simulink model "EVTOL_6DOF_Sim_Wrapper"  (R2025b)
settings: Solver=VariableStepAuto  StartTime=startTime  StopTime=stopTime  RelTol=1e-3
undefined symbols (not defined in the file): accel_mem_init, controller_mode, controller_sample_time, DiscIntNeverNeededParam, eul_init, gains, K_lqr_cruise, lla_init, MixMatrix, omega_init, pos_init, sat, sensor_accel_bias, sensor_accel_sigma, sensor_airdata_bias, sensor_airdata_sigma, sensor_att_bias, sensor_att_sigma, sensor_gps_posBias, sensor_gps_posSigma, sensor_gyro_bias, sensor_gyro_sigma, sensor_mag_bias, sensor_mag_sigma, sensor_magField_NED, sensor_sample_time, sensor_seed_accel, sensor_seed_airdata, sensor_seed_att, sensor_seed_gpsPos, sensor_seed_gyro, sensor_seed_mag, U_trim_lqr, useCMDs, V_mem_init, x_trim_lqr
settings Model: Creator=zbrown  LastModifiedBy=jacks

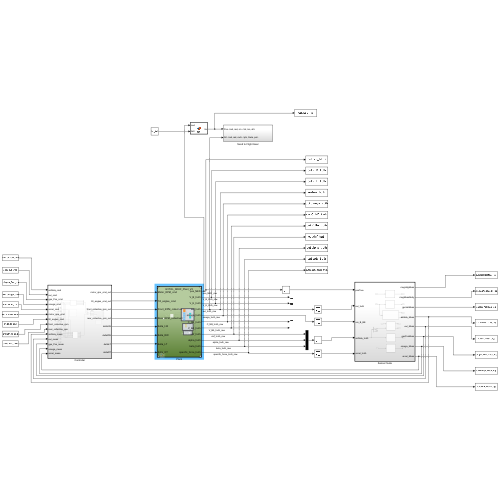
[thumbnail: Simulink's stored preview of the top-level diagram]
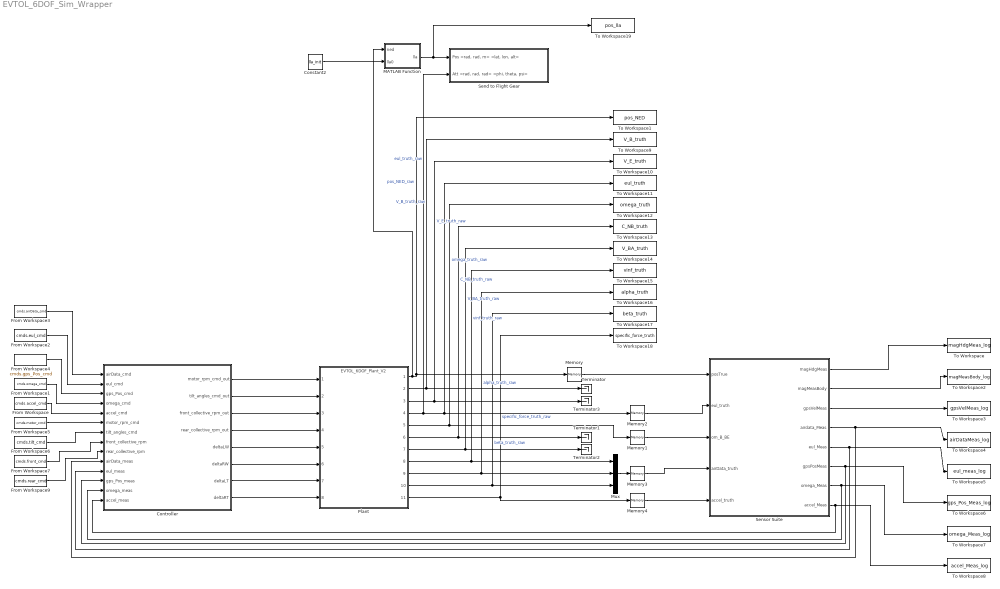
== system EVTOL_6DOF_Sim_Wrapper ==
  Constant2 : Constant  Value=lla_init
  Controller : Subsystem  TreatAsAtomicUnit=on  SystemSampleTime=controller_sample_time
  From Workspace : FromWorkspace  VariableName=cmds.accel_cmd
  From Workspace1 : FromWorkspace  VariableName=cmds.omega_cmd
  From Workspace2 : FromWorkspace  VariableName=cmds.eul_cmd
  From Workspace3 : FromWorkspace  VariableName=cmds.airData_cmd
  From Workspace4 : FromWorkspace  VariableName=cmds.gps_Pos_cmd
  From Workspace5 : FromWorkspace  VariableName=cmds.motor_cmd
  From Workspace6 : FromWorkspace  VariableName=cmds.tilt_cmd
  From Workspace7 : FromWorkspace  VariableName=cmds.front_cmd
  From Workspace9 : FromWorkspace  VariableName=cmds.rear_cmd
  MATLAB Function : MATLAB Function  TreatAsAtomicUnit=on
  Memory : Memory  InitialCondition=pos_init
  Memory1 : Memory  InitialCondition=omega_init
  Memory2 : Memory  InitialCondition=eul_init
  Memory3 : Memory  InitialCondition=V_mem_init
  Memory4 : Memory  InitialCondition=accel_mem_init
  Mux : Mux  Inputs=3
  Plant : ModelReference  ModelNameDialog=EVTOL_6DOF_Plant_V2.slx  SimulationMode=Normal  ModelReferenceVersion=1.34
  Send to Flight Gear : Subsystem
  Sensor Suite : Subsystem  TreatAsAtomicUnit=on  SystemSampleTime=sensor_sample_time
  Terminator{,1..3} (4 alike) : Terminator
  To Workspace : ToWorkspace  VariableName=magHdgMeas_log  SaveFormat=Structure With Time  SampleTime=-1
  To Workspace1 : ToWorkspace  VariableName=pos_NED  SaveFormat=Structure With Time  SampleTime=-1
  To Workspace10 : ToWorkspace  VariableName=V_E_truth  SaveFormat=Structure With Time  SampleTime=-1
  To Workspace11 : ToWorkspace  VariableName=eul_truth  SaveFormat=Structure With Time  SampleTime=-1
  To Workspace12 : ToWorkspace  VariableName=omega_truth  SaveFormat=Structure With Time  SampleTime=-1
  To Workspace13 : ToWorkspace  VariableName=C_NB_truth  SaveFormat=Structure With Time  SampleTime=-1
  To Workspace14 : ToWorkspace  VariableName=V_BA_truth  SaveFormat=Structure With Time  SampleTime=-1
  To Workspace15 : ToWorkspace  VariableName=vinf_truth  SaveFormat=Structure With Time  SampleTime=-1
  To Workspace16 : ToWorkspace  VariableName=alpha_truth  SaveFormat=Structure With Time  SampleTime=-1
  To Workspace17 : ToWorkspace  VariableName=beta_truth  SaveFormat=Structure With Time  SampleTime=-1
  To Workspace18 : ToWorkspace  VariableName=specific_force_truth  SaveFormat=Structure With Time  SampleTime=-1
  To Workspace19 : ToWorkspace  VariableName=pos_lla  SaveFormat=Structure With Time  SampleTime=-1
  To Workspace2 : ToWorkspace  VariableName=magMeasBody_log  SaveFormat=Structure With Time  SampleTime=-1
  To Workspace3 : ToWorkspace  VariableName=gpsVelMeas_log  SaveFormat=Structure With Time  SampleTime=-1
  To Workspace4 : ToWorkspace  VariableName=airDataMeas_log  SaveFormat=Structure With Time  SampleTime=-1
  To Workspace5 : ToWorkspace  VariableName=eul_meas_log  SaveFormat=Structure With Time  SampleTime=-1
  To Workspace6 : ToWorkspace  VariableName=gps_Pos_Meas_log  SaveFormat=Structure With Time  SampleTime=-1
  To Workspace7 : ToWorkspace  VariableName=omega_Meas_log  SaveFormat=Structure With Time  SampleTime=-1
  To Workspace8 : ToWorkspace  VariableName=accel_Meas_log  SaveFormat=Structure With Time  SampleTime=-1
  To Workspace9 : ToWorkspace  VariableName=V_B_truth  SaveFormat=Structure With Time  SampleTime=-1
  wires:
  Plant/1 -> MATLAB Function/1(ned), Memory/1, To Workspace1/1  "pos_NED_raw"
  Plant/2 -> Terminator/1, To Workspace9/1  "V_B_truth_raw"
  Plant/3 -> Terminator3/1, To Workspace10/1  "V_E_truth_raw"
  Plant/4 -> Send to Flight Gear/2("Att <rad, rad, rad> <phi, theta, psi>"), To Workspace11/1, Memory2/1  "eul_truth_raw"
  Plant/5 -> Memory1/1, To Workspace12/1  "omega_truth_raw"
  Plant/6 -> Terminator1/1, To Workspace13/1  "C_NB_truth_raw"
  Plant/7 -> Terminator2/1, To Workspace14/1  "V_BA_truth_raw"
  Plant/8 -> Mux/1, To Workspace15/1  "vinf_truth_raw"
  Plant/9 -> Mux/2, To Workspace16/1  "alpha_truth_raw"
  Plant/10 -> Mux/3, To Workspace17/1  "beta_truth_raw"
  Plant/11 -> Memory4/1, To Workspace18/1  "specific_force_truth_raw"
  MATLAB Function/1(lla) -> To Workspace19/1, Send to Flight Gear/1("Pos <rad, rad, m> <lat, lon, alt>")
  Constant2/1 -> MATLAB Function/2(lla0)
  Mux/1 -> Memory3/1
  Controller/5(deltaLW) -> Plant/5
  Controller/6(deltaRW) -> Plant/6
  Controller/7(deltaLT) -> Plant/7
  Controller/8(deltaRT) -> Plant/8
  Controller/4(rear_collective_rpm_out) -> Plant/4
  Controller/3(front_collective_rpm_out) -> Plant/3
  Controller/2(tilt_angles_cmd_out) -> Plant/2
  Controller/1(motor_rpm_cmd_out) -> Plant/1
  Sensor Suite/8(accel_Meas) -> Controller/14(accel_meas), To Workspace8/1
  Sensor Suite/7(omega_Meas) -> To Workspace7/1, Controller/13(omega_meas)
  Sensor Suite/6(gpsPosMeas) -> Controller/12(gps_Pos_meas), To Workspace6/1
  Sensor Suite/5(eul_Meas) -> Controller/11(eul_meas), To Workspace5/1
  Sensor Suite/4(airdata_Meas) -> Controller/10(airData_meas), To Workspace4/1
  From Workspace3/1 -> Controller/1(airData_cmd)
  From Workspace2/1 -> Controller/2(eul_cmd)
  From Workspace4/1 -> Controller/3(gps_Pos_cmd)
  From Workspace1/1 -> Controller/4(omega_cmd)
  From Workspace/1 -> Controller/5(accel_cmd)
  From Workspace5/1 -> Controller/6(motor_rpm_cmd)
  From Workspace6/1 -> Controller/7(tilt_angles_cmd)
  From Workspace7/1 -> Controller/8(front_collective_rpm)
  From Workspace9/1 -> Controller/9(rear_collective_rpm)
  Sensor Suite/1(magHdgMeas) -> To Workspace/1
  Sensor Suite/2(magMeasBody) -> To Workspace2/1
  Sensor Suite/3(gpsVelMeas) -> To Workspace3/1
  Memory/1 -> Sensor Suite/1(posTrue)
  Memory4/1 -> Sensor Suite/5(accel_truth)
  Memory3/1 -> Sensor Suite/4(airData_truth)
  Memory2/1 -> Sensor Suite/2(eul_truth)
  Memory1/1 -> Sensor Suite/3(om_B_BE)

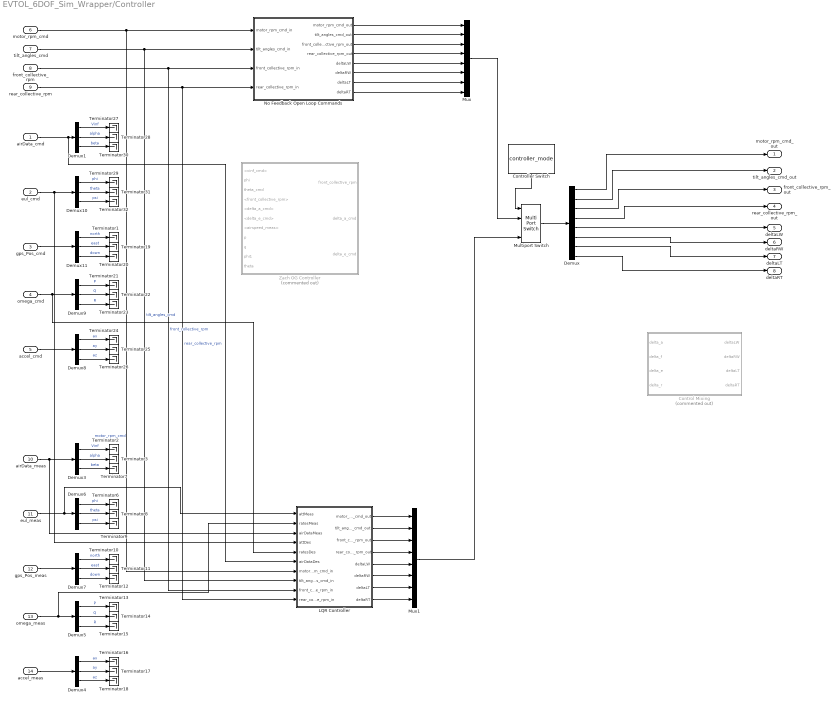
== system EVTOL_6DOF_Sim_Wrapper/Controller ==
  airData_cmd : Inport
  eul_cmd : Inport  Port=2
  gps_Pos_cmd : Inport  Port=3
  omega_cmd : Inport  Port=4
  accel_cmd : Inport  Port=5
  motor_rpm_cmd : Inport  Port=6
  tilt_angles_cmd : Inport  Port=7
  front_collective_rpm : Inport  Port=8
  rear_collective_rpm : Inport  Port=9
  airData_meas : Inport  Port=10
  eul_meas : Inport  Port=11
  gps_Pos_meas : Inport  Port=12
  omega_meas : Inport  Port=13
  accel_meas : Inport  Port=14
  Control Mixing : Subsystem  Commented=on
  Controller Switch : Constant  Value=controller_mode
  Demux : Demux  Outputs=8
  Demux{1,3..11} (10 alike) : Demux  Outputs=3
  LQR Controller : Subsystem
  Multiport Switch : MultiPortSwitch  SaturateOnIntegerOverflow=off  InputSameDT=off
  Mux : Mux  Inputs=8
  Mux1 : Mux  Inputs=8
  No Feedback Open Loop Commands : Subsystem
  Terminator{1..3,6..32} (30 alike) : Terminator
  Zach OG Controller : Subsystem  Commented=on
  motor_rpm_cmd_out : Outport
  tilt_angles_cmd_out : Outport  Port=2
  front_collective_rpm_out : Outport  Port=3
  rear_collective_rpm_out : Outport  Port=4
  deltaLW : Outport  Port=5
  deltaRW : Outport  Port=6
  deltaLT : Outport  Port=7
  deltaRT : Outport  Port=8
  wires:
  Demux11/2 -> Terminator19/1  "east"
  Demux6/3 -> Terminator9/1  "psi"
  Demux9/1 -> Terminator21/1  "P"
  motor_rpm_cmd/1 -> LQR Controller/7(motor_rpm_cmd_in), No Feedback Open Loop Commands/1(motor_rpm_cmd_in)  "motor_rpm_cmd"
  omega_cmd/1 -> LQR Controller/5(ratesDes), Demux9/1
  No Feedback Open Loop Commands/7(deltaLT) -> Mux/7
  Demux4/2 -> Terminator17/1  "ay"
  gps_Pos_cmd/1 -> Demux11/1
  Demux3/3 -> Terminator7/1  "beta"
  eul_meas/1 -> LQR Controller/1(attMeas), Demux6/1
  tilt_angles_cmd/1 -> LQR Controller/8(tilt_angles_cmd_in), No Feedback Open Loop Commands/2(tilt_angles_cmd_in)  "tilt_angles_cmd"
  Demux4/3 -> Terminator18/1  "az"
  Demux9/3 -> Terminator23/1  "R"
  airData_meas/1 -> LQR Controller/3(airDataMeas), Demux3/1
  Demux/2 -> tilt_angles_cmd_out/1
  Demux/4 -> rear_collective_rpm_out/1
  Demux8/1 -> Terminator24/1  "ax"
  Demux5/1 -> Terminator13/1  "P"
  Demux/1 -> motor_rpm_cmd_out/1
  No Feedback Open Loop Commands/6(deltaRW) -> Mux/6
  eul_cmd/1 -> LQR Controller/4(attDes), Demux10/1
  Demux3/2 -> Terminator3/1  "alpha"
  Demux9/2 -> Terminator22/1  "Q"
  Demux4/1 -> Terminator16/1  "ax"
  front_collective_rpm/1 -> LQR Controller/9(front_collective_rpm_in), No Feedback Open Loop Commands/3(front_collective_rpm_in)  "front_collective_rpm"
  Demux10/1 -> Terminator29/1  "phi"
  Demux8/3 -> Terminator26/1  "az"
  Demux7/1 -> Terminator10/1  "north"
  No Feedback Open Loop Commands/3(front_collective_rpm_out) -> Mux/3
  Demux6/1 -> Terminator6/1  "phi"
  Demux1/1 -> Terminator27/1  "Vinf"
  airData_cmd/1 -> LQR Controller/6(airDataDes), Demux1/1
  rear_collective_rpm/1 -> LQR Controller/10(rear_collective_rpm_in), No Feedback Open Loop Commands/4(rear_collective_rpm_in)  "rear_collective_rpm"
  Demux11/3 -> Terminator20/1  "down"
  Demux3/1 -> Terminator2/1  "Vinf"
  Demux6/2 -> Terminator8/1  "theta"
  Demux10/3 -> Terminator32/1  "psi"
  Demux5/3 -> Terminator15/1  "R"
  Mux/1 -> Multiport Switch/2
  No Feedback Open Loop Commands/2(tilt_angles_cmd_out) -> Mux/2
  accel_meas/1 -> Demux4/1
  No Feedback Open Loop Commands/4(rear_collective_rpm_out) -> Mux/4
  Demux5/2 -> Terminator14/1  "Q"
  Demux11/1 -> Terminator1/1  "north"
  Demux8/2 -> Terminator25/1  "ay"
  Demux1/3 -> Terminator30/1  "beta"
  gps_Pos_meas/1 -> Demux7/1
  Demux7/2 -> Terminator11/1  "east"
  Demux/3 -> front_collective_rpm_out/1
  Demux10/2 -> Terminator31/1  "theta"
  No Feedback Open Loop Commands/1(motor_rpm_cmd_out) -> Mux/1
  omega_meas/1 -> LQR Controller/2(ratesMeas), Demux5/1
  Demux7/3 -> Terminator12/1  "down"
  accel_cmd/1 -> Demux8/1
  No Feedback Open Loop Commands/8(deltaRT) -> Mux/8
  Multiport Switch/1 -> Demux/1
  No Feedback Open Loop Commands/5(deltaLW) -> Mux/5
  Demux1/2 -> Terminator28/1  "alpha"
  Controller Switch/1 -> Multiport Switch/1
  Demux/5 -> deltaLW/1
  Demux/6 -> deltaRW/1
  Demux/7 -> deltaLT/1
  Demux/8 -> deltaRT/1
  LQR Controller/7(deltaLT) -> Mux1/7
  LQR Controller/5(deltaLW) -> Mux1/5
  LQR Controller/4(rear_collective_rpm_out) -> Mux1/4
  LQR Controller/3(front_collective_rpm_out) -> Mux1/3
  LQR Controller/1(motor_rpm_cmd_out) -> Mux1/1
  LQR Controller/2(tilt_angles_cmd_out) -> Mux1/2
  LQR Controller/6(deltaRW) -> Mux1/6
  LQR Controller/8(deltaRT) -> Mux1/8
  Mux1/1 -> Multiport Switch/4

== system EVTOL_6DOF_Sim_Wrapper/Send to Flight Gear ==
  "Pos <rad, rad, m> <lat, lon, alt>" : Inport
  "Att <rad, rad, rad> <phi, theta, psi>" : Inport  Port=2
  S-Function : S-Function  FunctionName=sfun_FlightGearSender  Parameters=stepTime, '127.0.0.1', 5502  SFunctionDeploymentMode=off  EnableBusSupport=off
  wires:
  "Pos <rad, rad, m> <lat, lon, alt>"/1 -> S-Function/1
  "Att <rad, rad, rad> <phi, theta, psi>"/1 -> S-Function/2

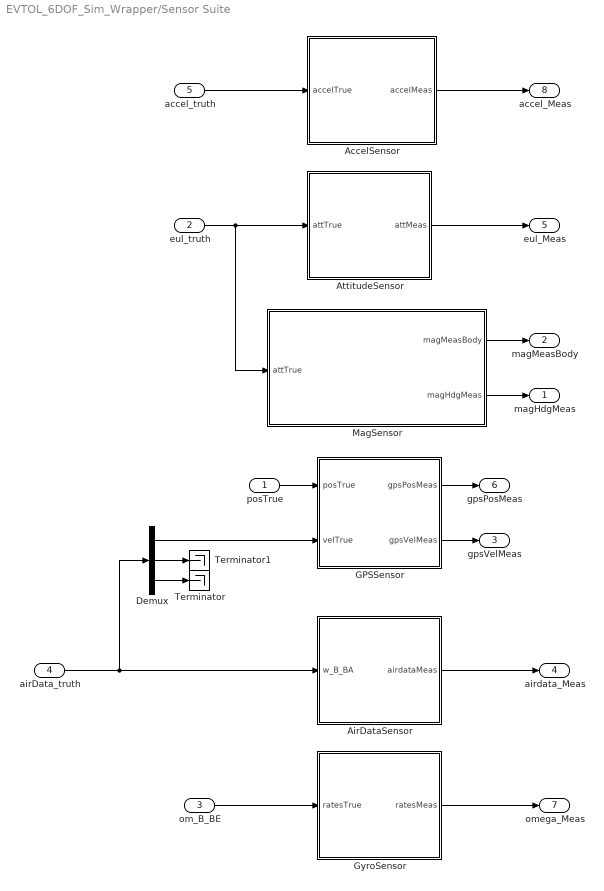
== system EVTOL_6DOF_Sim_Wrapper/Sensor Suite ==
  posTrue : Inport
  eul_truth : Inport  Port=2
  om_B_BE : Inport  Port=3
  airData_truth : Inport  Port=4
  accel_truth : Inport  Port=5
  AccelSensor : Subsystem
  AirDataSensor : Subsystem
  AttitudeSensor : Subsystem
  Demux : Demux  Outputs=3
  GPSSensor : Subsystem
  GyroSensor : Subsystem
  MagSensor : Subsystem
  Terminator : Terminator
  Terminator1 : Terminator
  magHdgMeas : Outport
  magMeasBody : Outport  Port=2
  gpsVelMeas : Outport  Port=3
  airdata_Meas : Outport  Port=4
  eul_Meas : Outport  Port=5  VectorParamsAs1DForOutWhenUnconnected=off
  gpsPosMeas : Outport  Port=6
  omega_Meas : Outport  Port=7  VectorParamsAs1DForOutWhenUnconnected=off
  accel_Meas : Outport  Port=8  VectorParamsAs1DForOutWhenUnconnected=off
  wires:
  GyroSensor/1(ratesMeas) -> omega_Meas/1
  eul_truth/1 -> AttitudeSensor/1(attTrue), MagSensor/1(attTrue)
  AccelSensor/1(accelMeas) -> accel_Meas/1
  posTrue/1 -> GPSSensor/1(posTrue)
  AirDataSensor/1(airdataMeas) -> airdata_Meas/1
  AttitudeSensor/1(attMeas) -> eul_Meas/1
  om_B_BE/1 -> GyroSensor/1(ratesTrue)
  GPSSensor/2(gpsVelMeas) -> gpsVelMeas/1
  MagSensor/2(magHdgMeas) -> magHdgMeas/1
  accel_truth/1 -> AccelSensor/1(accelTrue)
  GPSSensor/1(gpsPosMeas) -> gpsPosMeas/1
  MagSensor/1(magMeasBody) -> magMeasBody/1
  airData_truth/1 -> Demux/1, AirDataSensor/1(w_B_BA)
  Demux/1 -> GPSSensor/2(velTrue)
  Demux/2 -> Terminator1/1
  Demux/3 -> Terminator/1

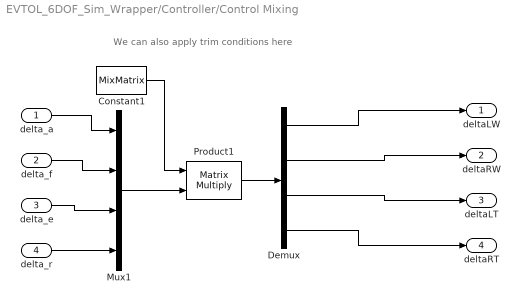
== system EVTOL_6DOF_Sim_Wrapper/Controller/Control Mixing ==
  note: We can also apply trim conditions here
  delta_a : Inport
  delta_f : Inport  Port=2
  delta_e : Inport  Port=3
  delta_r : Inport  Port=4
  Constant1 : Constant  Value=MixMatrix
  Demux : Demux
  Mux1 : Mux
  Product1 : Product  Multiplication=Matrix(*)
  deltaLW : Outport
  deltaRW : Outport  Port=2
  deltaLT : Outport  Port=3
  deltaRT : Outport  Port=4
  wires:
  delta_a/1 -> Mux1/1
  Demux/1 -> deltaLW/1
  delta_f/1 -> Mux1/2
  Mux1/1 -> Product1/2
  delta_e/1 -> Mux1/3
  Constant1/1 -> Product1/1
  delta_r/1 -> Mux1/4
  Demux/2 -> deltaRW/1
  Product1/1 -> Demux/1
  Demux/3 -> deltaLT/1
  Demux/4 -> deltaRT/1

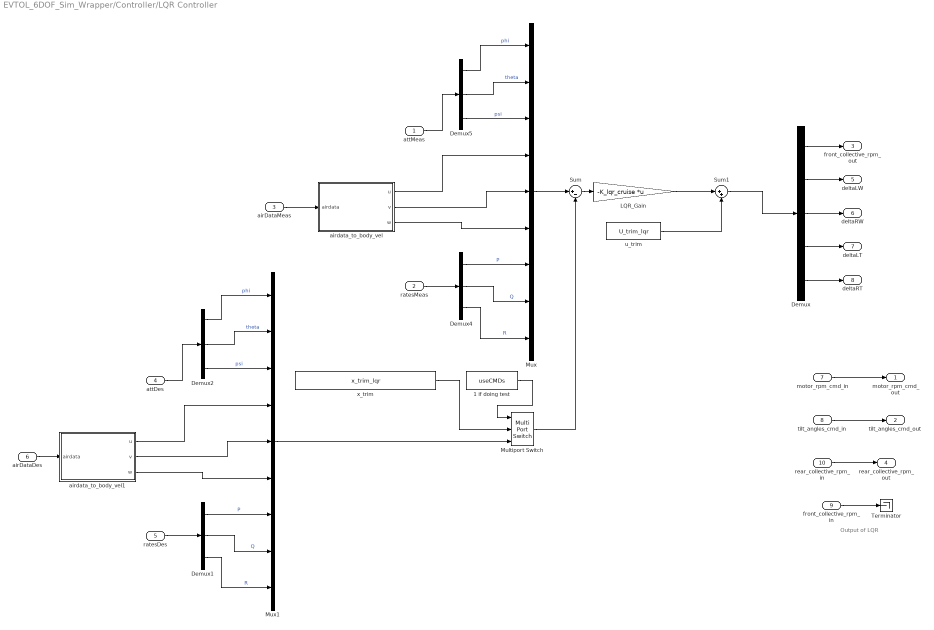
== system EVTOL_6DOF_Sim_Wrapper/Controller/LQR Controller ==
  note: Output of LQR
  attMeas : Inport
  ratesMeas : Inport  Port=2
  airDataMeas : Inport  Port=3
  attDes : Inport  Port=4
  ratesDes : Inport  Port=5
  airDataDes : Inport  Port=6
  motor_rpm_cmd_in : Inport  Port=7
  tilt_angles_cmd_in : Inport  Port=8
  front_collective_rpm_in : Inport  Port=9
  rear_collective_rpm_in : Inport  Port=10
  1 if doing test : Constant  Value=useCMDs
  Demux : Demux  Outputs=5
  Demux{1..2,4..5} (4 alike) : Demux  Outputs=3
  LQR_Gain : Gain  Gain=-K_lqr_cruise  Multiplication=Matrix(K*u)
  Multiport Switch : MultiPortSwitch  Inputs=2  SaturateOnIntegerOverflow=off  InputSameDT=off
  Mux : Mux  Inputs=9
  Mux1 : Mux  Inputs=9
  Sum : Sum  Inputs=|+-
  Sum1 : Sum  Inputs=|++
  Terminator : Terminator
  airdata_to_body_vel : MATLAB Function  TreatAsAtomicUnit=on
  airdata_to_body_vel1 : MATLAB Function  TreatAsAtomicUnit=on
  u_trim : Constant  Value=U_trim_lqr
  x_trim : Constant  Value=x_trim_lqr
  motor_rpm_cmd_out : Outport
  tilt_angles_cmd_out : Outport  Port=2
  front_collective_rpm_out : Outport  Port=3
  rear_collective_rpm_out : Outport  Port=4
  deltaLW : Outport  Port=5
  deltaRW : Outport  Port=6
  deltaLT : Outport  Port=7
  deltaRT : Outport  Port=8
  wires:
  Demux/4 -> deltaLT/1
  attMeas/1 -> Demux5/1
  airDataMeas/1 -> airdata_to_body_vel/1(airdata)
  ratesMeas/1 -> Demux4/1
  Demux5/2 -> Mux/2  "theta"
  Demux5/1 -> Mux/1  "phi"
  Demux5/3 -> Mux/3  "psi"
  u_trim/1 -> Sum1/2
  Demux4/1 -> Mux/7  "P"
  Demux4/3 -> Mux/9  "R"
  Demux4/2 -> Mux/8  "Q"
  Mux/1 -> Sum/1
  Sum/1 -> LQR_Gain/1
  LQR_Gain/1 -> Sum1/1
  Sum1/1 -> Demux/1
  Demux/1 -> front_collective_rpm_out/1
  Demux/2 -> deltaLW/1
  Demux/3 -> deltaRW/1
  airdata_to_body_vel/1(u) -> Mux/4
  airdata_to_body_vel/2(v) -> Mux/5
  airdata_to_body_vel/3(w) -> Mux/6
  airdata_to_body_vel1/3(w) -> Mux1/6
  airdata_to_body_vel1/2(v) -> Mux1/5
  ratesDes/1 -> Demux1/1
  attDes/1 -> Demux2/1
  Demux1/3 -> Mux1/9  "R"
  Demux1/2 -> Mux1/8  "Q"
  Demux2/3 -> Mux1/3  "psi"
  Demux2/1 -> Mux1/1  "phi"
  Demux2/2 -> Mux1/2  "theta"
  airdata_to_body_vel1/1(u) -> Mux1/4
  Demux1/1 -> Mux1/7  "P"
  airDataDes/1 -> airdata_to_body_vel1/1(airdata)
  Multiport Switch/1 -> Sum/2
  1 if doing test/1 -> Multiport Switch/1
  x_trim/1 -> Multiport Switch/2
  Mux1/1 -> Multiport Switch/3
  Demux/5 -> deltaRT/1
  motor_rpm_cmd_in/1 -> motor_rpm_cmd_out/1
  tilt_angles_cmd_in/1 -> tilt_angles_cmd_out/1
  rear_collective_rpm_in/1 -> rear_collective_rpm_out/1
  front_collective_rpm_in/1 -> Terminator/1

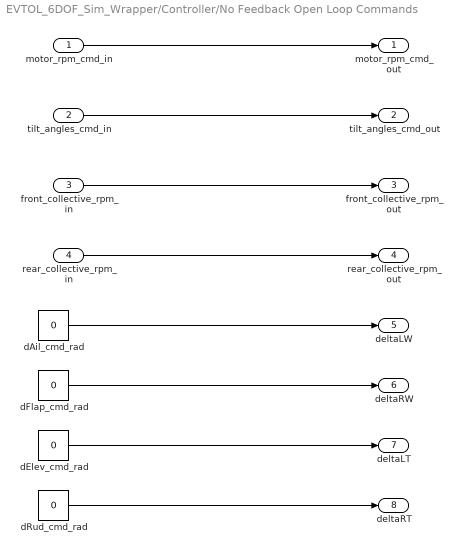
== system EVTOL_6DOF_Sim_Wrapper/Controller/No Feedback Open Loop Commands ==
  motor_rpm_cmd_in : Inport
  tilt_angles_cmd_in : Inport  Port=2
  front_collective_rpm_in : Inport  Port=3
  rear_collective_rpm_in : Inport  Port=4
  dAil_cmd_rad : Constant  Value=0
  dElev_cmd_rad : Constant  Value=0
  dFlap_cmd_rad : Constant  Value=0
  dRud_cmd_rad : Constant  Value=0
  motor_rpm_cmd_out : Outport
  tilt_angles_cmd_out : Outport  Port=2
  front_collective_rpm_out : Outport  Port=3
  rear_collective_rpm_out : Outport  Port=4
  deltaLW : Outport  Port=5
  deltaRW : Outport  Port=6
  deltaLT : Outport  Port=7
  deltaRT : Outport  Port=8
  wires:
  dElev_cmd_rad/1 -> deltaLT/1
  dAil_cmd_rad/1 -> deltaLW/1
  front_collective_rpm_in/1 -> front_collective_rpm_out/1
  rear_collective_rpm_in/1 -> rear_collective_rpm_out/1
  tilt_angles_cmd_in/1 -> tilt_angles_cmd_out/1
  dFlap_cmd_rad/1 -> deltaRW/1
  motor_rpm_cmd_in/1 -> motor_rpm_cmd_out/1
  dRud_cmd_rad/1 -> deltaRT/1

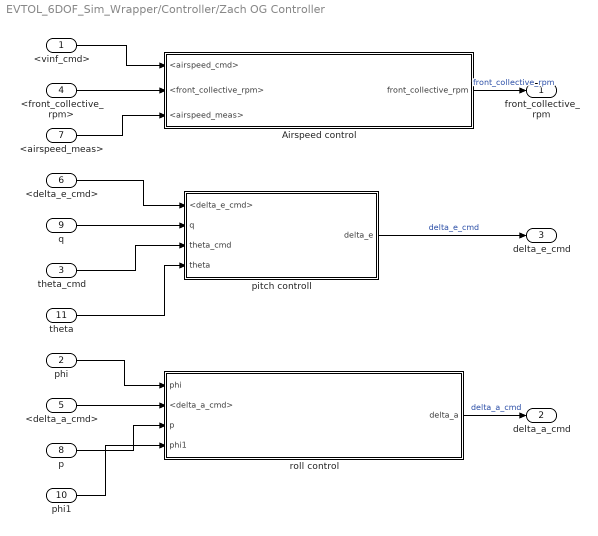
== system EVTOL_6DOF_Sim_Wrapper/Controller/Zach OG Controller ==
  <vinf_cmd> : Inport
  phi : Inport  Port=2
  theta_cmd : Inport  Port=3
  <front_collective_rpm> : Inport  Port=4
  <delta_a_cmd> : Inport  Port=5
  <delta_e_cmd> : Inport  Port=6
  <airspeed_meas> : Inport  Port=7
  p : Inport  Port=8
  q : Inport  Port=9
  phi1 : Inport  Port=10
  theta : Inport  Port=11
  Airspeed control : Subsystem
  pitch controll : Subsystem
  roll control : Subsystem
  front_collective_rpm : Outport
  delta_a_cmd : Outport  Port=2
  delta_e_cmd : Outport  Port=3
  wires:
  <vinf_cmd>/1 -> Airspeed control/1(<airspeed_cmd>)
  <front_collective_rpm>/1 -> Airspeed control/2(<front_collective_rpm>)
  theta/1 -> pitch controll/4(theta)
  <airspeed_meas>/1 -> Airspeed control/3(<airspeed_meas>)
  <delta_e_cmd>/1 -> pitch controll/1(<delta_e_cmd>)
  q/1 -> pitch controll/2(q)
  theta_cmd/1 -> pitch controll/3(theta_cmd)
  phi/1 -> roll control/1(phi)
  <delta_a_cmd>/1 -> roll control/2(<delta_a_cmd>)
  p/1 -> roll control/3(p)
  phi1/1 -> roll control/4(phi1)
  Airspeed control/1(front_collective_rpm) -> front_collective_rpm/1  "front_collective_rpm"
  pitch controll/1(delta_e) -> delta_e_cmd/1  "delta_e_cmd"
  roll control/1(delta_a) -> delta_a_cmd/1  "delta_a_cmd"

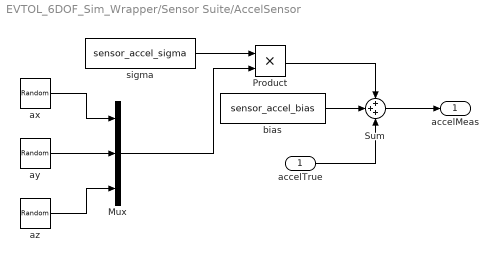
== system EVTOL_6DOF_Sim_Wrapper/Sensor Suite/AccelSensor ==
  accelTrue : Inport
  Mux : Mux  Inputs=3
  Product : Product
  Sum : Sum  Inputs=+++
  ax : RandomNumber  Seed=sensor_seed_accel  SampleTime=sensor_sample_time
  ay : RandomNumber  Seed=sensor_seed_accel + 1  SampleTime=sensor_sample_time
  az : RandomNumber  Seed=sensor_seed_accel + 2  SampleTime=sensor_sample_time
  bias : Constant  Value=sensor_accel_bias
  sigma : Constant  Value=sensor_accel_sigma
  accelMeas : Outport
  wires:
  ax/1 -> Mux/1
  accelTrue/1 -> Sum/3
  ay/1 -> Mux/2
  az/1 -> Mux/3
  sigma/1 -> Product/1
  bias/1 -> Sum/2
  Mux/1 -> Product/2
  Product/1 -> Sum/1
  Sum/1 -> accelMeas/1

== system EVTOL_6DOF_Sim_Wrapper/Sensor Suite/AirDataSensor ==
  w_B_BA : Inport
  Mux : Mux  Inputs=3
  Product : Product
  Sum : Sum  Inputs=+++
  Vinf_rnd : RandomNumber  Seed=sensor_seed_airdata  SampleTime=sensor_sample_time
  alpha_rnd : RandomNumber  Seed=sensor_seed_airdata + 1  SampleTime=sensor_sample_time
  beta_rnd : RandomNumber  Seed=sensor_seed_airdata + 2  SampleTime=sensor_sample_time
  bias : Constant  Value=sensor_airdata_bias
  sigma : Constant  Value=sensor_airdata_sigma
  airdataMeas : Outport
  wires:
  Vinf_rnd/1 -> Mux/1
  w_B_BA/1 -> Sum/3
  Product/1 -> Sum/1
  alpha_rnd/1 -> Mux/2
  beta_rnd/1 -> Mux/3
  sigma/1 -> Product/1
  Mux/1 -> Product/2
  bias/1 -> Sum/2
  Sum/1 -> airdataMeas/1

== system EVTOL_6DOF_Sim_Wrapper/Sensor Suite/AttitudeSensor ==
  attTrue : Inport
  Mux : Mux  Inputs=3
  Product : Product
  Sum : Sum  Inputs=+++
  bias : Constant  Value=sensor_att_bias
  phi : RandomNumber  Seed=sensor_seed_att  SampleTime=sensor_sample_time
  psi : RandomNumber  Seed=sensor_seed_att + 2  SampleTime=sensor_sample_time
  sigma : Constant  Value=sensor_att_sigma
  theta : RandomNumber  Seed=sensor_seed_att + 1  SampleTime=sensor_sample_time
  attMeas : Outport
  wires:
  attTrue/1 -> Sum/3
  phi/1 -> Mux/1
  theta/1 -> Mux/2
  Product/1 -> Sum/1
  psi/1 -> Mux/3
  Mux/1 -> Product/2
  sigma/1 -> Product/1
  bias/1 -> Sum/2
  Sum/1 -> attMeas/1

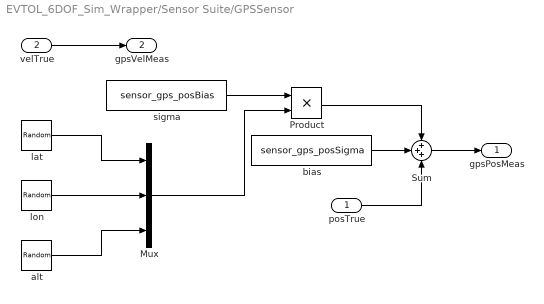
== system EVTOL_6DOF_Sim_Wrapper/Sensor Suite/GPSSensor ==
  posTrue : Inport
  velTrue : Inport  Port=2
  Mux : Mux  Inputs=3
  Product : Product
  Sum : Sum  Inputs=+++
  alt : RandomNumber  Seed=sensor_seed_gpsPos + 2  SampleTime=sensor_sample_time
  bias : Constant  Value=sensor_gps_posSigma
  lat : RandomNumber  Seed=sensor_seed_gpsPos  SampleTime=sensor_sample_time
  lon : RandomNumber  Seed=sensor_seed_gpsPos + 1  SampleTime=sensor_sample_time
  sigma : Constant  Value=sensor_gps_posBias
  gpsPosMeas : Outport
  gpsVelMeas : Outport  Port=2
  wires:
  lat/1 -> Mux/1
  bias/1 -> Sum/2
  velTrue/1 -> gpsVelMeas/1
  lon/1 -> Mux/2
  sigma/1 -> Product/1
  Sum/1 -> gpsPosMeas/1
  alt/1 -> Mux/3
  Mux/1 -> Product/2
  Product/1 -> Sum/1
  posTrue/1 -> Sum/3

== system EVTOL_6DOF_Sim_Wrapper/Sensor Suite/GyroSensor ==
  ratesTrue : Inport
  Mux : Mux  Inputs=3
  P : RandomNumber  Seed=sensor_seed_gyro  SampleTime=sensor_sample_time
  Product : Product
  Q : RandomNumber  Seed=sensor_seed_gyro + 1  SampleTime=sensor_sample_time
  R : RandomNumber  Seed=sensor_seed_gyro + 2  SampleTime=sensor_sample_time
  Sum : Sum  Inputs=+++
  bias : Constant  Value=sensor_gyro_bias
  sigma : Constant  Value=sensor_gyro_sigma
  ratesMeas : Outport
  wires:
  P/1 -> Mux/1
  Q/1 -> Mux/2
  Product/1 -> Sum/1
  R/1 -> Mux/3
  sigma/1 -> Product/1
  Mux/1 -> Product/2
  Sum/1 -> ratesMeas/1
  bias/1 -> Sum/2
  ratesTrue/1 -> Sum/3

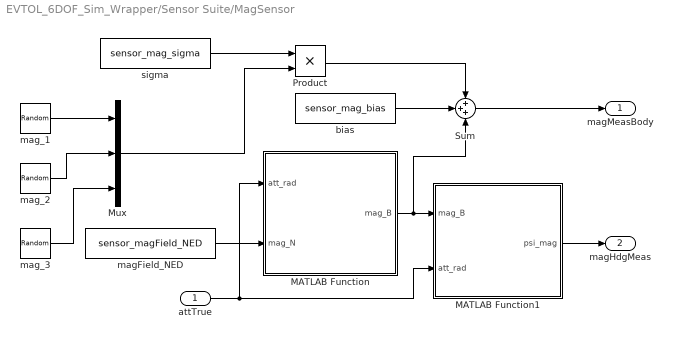
== system EVTOL_6DOF_Sim_Wrapper/Sensor Suite/MagSensor ==
  attTrue : Inport
  MATLAB Function : MATLAB Function  TreatAsAtomicUnit=on
  MATLAB Function1 : MATLAB Function  TreatAsAtomicUnit=on
  Mux : Mux  Inputs=3
  Product : Product
  Sum : Sum  Inputs=+++
  bias : Constant  Value=sensor_mag_bias
  magField_NED : Constant  Value=sensor_magField_NED
  mag_1 : RandomNumber  Seed=sensor_seed_mag  SampleTime=sensor_sample_time
  mag_2 : RandomNumber  Seed=sensor_seed_mag + 1  SampleTime=sensor_sample_time
  mag_3 : RandomNumber  Seed=sensor_seed_mag + 2  SampleTime=sensor_sample_time
  sigma : Constant  Value=sensor_mag_sigma
  magMeasBody : Outport
  magHdgMeas : Outport  Port=2
  wires:
  mag_1/1 -> Mux/1
  Mux/1 -> Product/2
  mag_2/1 -> Mux/2
  mag_3/1 -> Mux/3
  Product/1 -> Sum/1
  sigma/1 -> Product/1
  magField_NED/1 -> MATLAB Function/2(mag_N)
  attTrue/1 -> MATLAB Function1/2(att_rad), MATLAB Function/1(att_rad)
  bias/1 -> Sum/2
  MATLAB Function/1(mag_B) -> Sum/3, MATLAB Function1/1(mag_B)
  Sum/1 -> magMeasBody/1
  MATLAB Function1/1(psi_mag) -> magHdgMeas/1

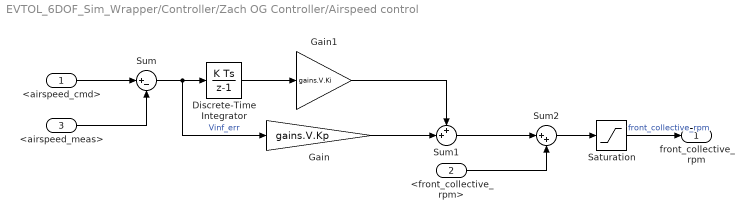
== system EVTOL_6DOF_Sim_Wrapper/Controller/Zach OG Controller/Airspeed control ==
  <airspeed_cmd> : Inport
  <front_collective_rpm> : Inport  Port=2
  <airspeed_meas> : Inport  Port=3
  Discrete-Time Integrator : DiscreteIntegrator  SampleTime=controller_sample_time  LimitOutput=on  UpperSaturationLimit=5000  LowerSaturationLimit=-5000  ICPrevOutput=DiscIntNeverNeededParam  ICPrevScaledInput=DiscIntNeverNeededParam
  Gain : Gain  Gain=gains.V.Kp
  Gain1 : Gain  Gain=gains.V.Ki
  Saturation : Saturate  UpperLimit=sat.frontcollective.high  LowerLimit=sat.frontcollective.low
  Sum : Sum  Inputs=|+-
  Sum1 : Sum  Inputs=++|
  Sum2 : Sum  Inputs=|++
  front_collective_rpm : Outport
  wires:
  <front_collective_rpm>/1 -> Sum2/2
  <airspeed_meas>/1 -> Sum/2
  <airspeed_cmd>/1 -> Sum/1
  Saturation/1 -> front_collective_rpm/1  "front_collective_rpm"
  Sum1/1 -> Sum2/1
  Gain/1 -> Sum1/2
  Gain1/1 -> Sum1/1
  Discrete-Time Integrator/1 -> Gain1/1
  Sum2/1 -> Saturation/1
  Sum/1 -> Gain/1, Discrete-Time Integrator/1  "Vinf_err"

== system EVTOL_6DOF_Sim_Wrapper/Controller/Zach OG Controller/pitch controll ==
  <delta_e_cmd> : Inport
  q : Inport  Port=2
  theta_cmd : Inport  Port=3
  theta : Inport  Port=4
  Gain1 : Gain  Gain=gains.theta.Kd
  Gain2 : Gain  Gain=gains.theta.Kp
  Sum : Sum  Inputs=++-
  Sum1 : Sum  Inputs=|+-
  delta_e : Outport
  wires:
  q/1 -> Gain1/1
  <delta_e_cmd>/1 -> Sum/1
  Sum/1 -> delta_e/1  "delta_e"
  Gain1/1 -> Sum/2
  Gain2/1 -> Sum/3
  theta/1 -> Sum1/2
  theta_cmd/1 -> Sum1/1
  Sum1/1 -> Gain2/1  "theta_err"

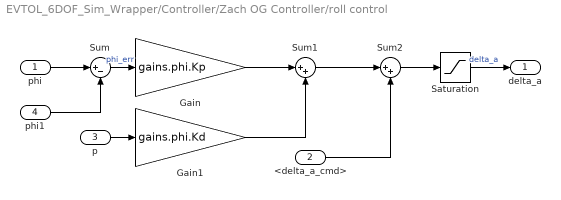
== system EVTOL_6DOF_Sim_Wrapper/Controller/Zach OG Controller/roll control ==
  phi : Inport
  <delta_a_cmd> : Inport  Port=2
  p : Inport  Port=3
  phi1 : Inport  Port=4
  Gain : Gain  Gain=gains.phi.Kp
  Gain1 : Gain  Gain=gains.phi.Kd
  Saturation : Saturate  UpperLimit=sat.delta_a.high  LowerLimit=sat.delta_a.low
  Sum : Sum  Inputs=|+-
  Sum1 : Sum  Inputs=|++
  Sum2 : Sum  Inputs=|++
  delta_a : Outport
  wires:
  <delta_a_cmd>/1 -> Sum2/2
  p/1 -> Gain1/1
  phi/1 -> Sum/1
  Gain1/1 -> Sum1/2
  Gain/1 -> Sum1/1
  Sum/1 -> Gain/1  "phi_err"
  phi1/1 -> Sum/2
  Sum1/1 -> Sum2/1
  Sum2/1 -> Saturation/1
  Saturation/1 -> delta_a/1  "delta_a"

== matlab function EVTOL_6DOF_Sim_Wrapper/Controller/LQR Controller/airdata_to_body_vel ==
  data: airdata input; u output; v output; w output
function [u, v, w] = airdata_to_body_vel(airdata)
    % Extract variables for readability
    V_inf = airdata(1);
    alpha = airdata(2);
    beta  = airdata(3);
    
    % Compute body-frame velocities
    u = V_inf * cos(alpha) * cos(beta);
    v = V_inf * sin(beta);
    w = V_inf * sin(alpha) * cos(beta);
end

== matlab function EVTOL_6DOF_Sim_Wrapper/Controller/LQR Controller/airdata_to_body_vel1 ==
  data: airdata input; u output; v output; w output
function [u, v, w] = airdata_to_body_vel(airdata)
    % Extract variables for readability
    V_inf = airdata(1);
    alpha = airdata(2);
    beta  = airdata(3);
    
    % Compute body-frame velocities
    u = V_inf * cos(alpha) * cos(beta);
    v = V_inf * sin(beta);
    w = V_inf * sin(alpha) * cos(beta);
end

== matlab function EVTOL_6DOF_Sim_Wrapper/Sensor Suite/MagSensor/MATLAB Function ==
  data: att_rad input; mag_B output; mag_N input
function mag_B = magField_NED_2_Body(att_rad, mag_N)
% Rotate the local magnetic field from NED into body axes.
% This keeps the model simple and gives you a raw 3-axis mag output that
% you can use later for heading estimation.

phi = att_rad(1);
theta = att_rad(2);
psi = att_rad(3);

cphi = cos(phi);
sphi = sin(phi);
cth = cos(theta);
sth = sin(theta);
cpsi = cos(psi);
spsi = sin(psi);

C_BN = [ cth*cpsi,                    cth*spsi,                   -sth;
         sphi*sth*cpsi-cphi*spsi,    sphi*sth*spsi+cphi*cpsi,    sphi*cth;
         cphi*sth*cpsi+sphi*spsi,    cphi*sth*spsi-sphi*cpsi,    cphi*cth ];

mag_B = C_BN * mag_N;

== matlab function EVTOL_6DOF_Sim_Wrapper/Sensor Suite/MagSensor/MATLAB Function1 ==
  data: mag_B input; psi_mag output; att_rad input
function psi_mag = derive_heading(mag_B, att_rad)
% Tilt-compensated heading estimate from a body-frame magnetometer and
% measured roll/pitch.

phi = att_rad(1);
theta = att_rad(2);

mx = mag_B(1);
my = mag_B(2);
mz = mag_B(3);

cphi = cos(phi);
sphi = sin(phi);
cth = cos(theta);
sth = sin(theta);

Xh = mx * cth + my * sphi * sth + mz * cphi * sth;
Yh = my * cphi - mz * sphi;

psi_mag = atan2(Yh, Xh);

== matlab function EVTOL_6DOF_Sim_Wrapper/MATLAB Function ==
  data: ned input; lla output; lla0 input
function lla  = fcn(ned, lla0)
% ned: 3-element vector [north, east, down] in meters
% lla0: 3-element vector [lat, lon, alt] origin in [deg, deg, m]
ned = ned';
lla0 = lla0';

lla = ned2lla(ned, lla0, 'flat');
end
